simulink model "ceshi20210729"  (R2016b)
settings: Solver=ode4  StartTime=0.0  StopTime=10.0  FixedStep=0.01  RelTol=1e-3
undefined symbols (not defined in the file): serial
libraries: instrumentlib x2
settings Model: Creator=lenovo  LastModifiedBy=lenovo

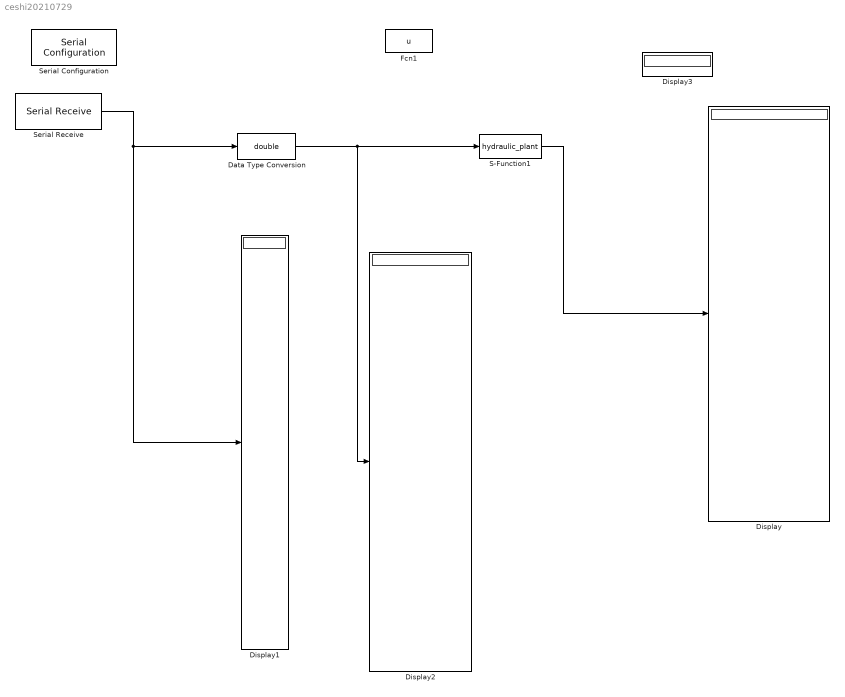
== system ceshi20210729 ==
  Data Type Conversion : DataTypeConversion  OutDataTypeStr=double
  Display{,1..3} (4 alike) : Display
      Display1 settings: Format=hex (Stored Integer)
  Fcn1 : Fcn  Expr=u
  S-Function1 : S-Function  FunctionName=hydraulic_plant  SFunctionDeploymentMode=off  EnableBusSupport=off
  Serial Configuration : instrumentlib/Serial Configuration  Priority=-200000  ComPortMenu=COM4  ComPort=COM4  ObjConstructor=serial('COM4');  BaudRate=115200  DataBits=8  Parity=none  StopBits=1  FlowControl=none  Timeout=10  ByteOrder=LittleEndian
  Serial Receive : instrumentlib/Serial Receive  ComPortMenu=COM4  ComPort=COM4  ObjConstructor=serial('COM4');  Terminator=<none>  DataSize="[1  29]"  DataType=uint8  EnableBlockingMode=on  ActionDataUnavailable=Output last received value  CustomValue=0  SampleTime=0.01
  wires:
  Serial Receive/1 -> Display1/1, Data Type Conversion/1
  Data Type Conversion/1 -> S-Function1/1, Display2/1
  S-Function1/1 -> Display/1
